simulink library "coolantFlowSwitch_lib"  (R2025a)
settings: Solver=VariableStepAuto  StartTime=0.0  StopTime=10.0  RelTol=1e-3
settings Model: Creator=mbhattu  LastModifiedBy=mbhattu

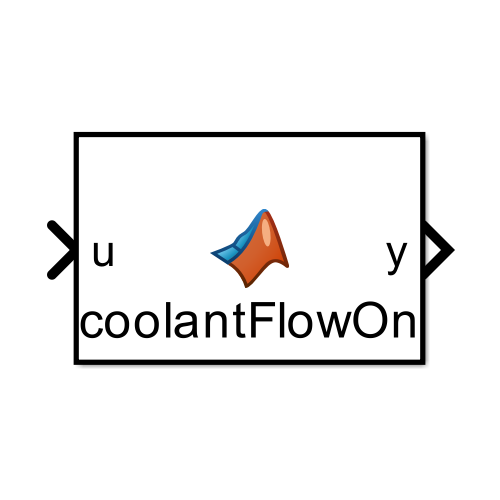
[thumbnail: Simulink's stored preview of the top-level diagram]
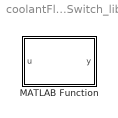
== system coolantFlowSwitch_lib ==
  MATLAB Function : MATLAB Function  TreatAsAtomicUnit=on

== matlab function coolantFlowSwitch_lib/MATLAB Function ==
  data: u input; y output
function y = coolantFlowOn(u)

y = double(u<-50);
